simulink model "Standalone_SpeedControl"  (R2023b)
settings: Solver=FixedStepAuto  StartTime=0.0  StopTime=Inf  RelTol=1e-3  EnableMultiTasking=on
undefined symbols (not defined in the file): SensorCurrent_VoltAtZero, SensorCurrent_VoltPerAmp
libraries: mcbpositiondecoderlib x1
settings Model: DataDictionary=Data_GeneralDefinition.sldd  SimulationMode=external  ExtModeTrigDuration=20  Creator=rodri  LastModifiedBy=rodri
settings OptimizationCC: DefaultUnderspecifiedDataType=single  EnhancedBackFolding=on  PassReuseOutputArgsAs=Individual arguments  MaxStackSize=1024  OptimizeBlockOrder=speed  DifferentSizesBufferReuse=on  EfficientTunableParamExpr=on
settings DebuggingCC: ParameterTunabilityLossMsg=error
settings HardwareCC: ProdBitPerChar=16  ProdBitPerInt=16  ProdBitPerPointer=32  ProdBitPerSizeT=32  ProdBitPerPtrDiffT=32  ProdLargestAtomicInteger=Integer  ProdLargestAtomicFloat=None  ProdWordSize=16  ProdLongLongMode=on  ProdHWDeviceType=Texas Instruments->C2000  HardwareBoardFeatureSet=SoCBlockset
settings ModelReferenceCC: EnableParallelModelReferenceBuilds=on  ModelReferenceNumInstancesAllowed=Single
settings SFSimCC: MATLABDynamicMemAlloc=off
settings RTWCC: Description=Embedded Coder  SystemTargetFile=ert.tlc  HardwareBoard=TI Piccolo F28069M LaunchPad  TemplateMakefile=ert_default_tmf  Toolchain=Texas Instruments Code Composer Studio (C2000)  CodeProfilingSaveOptions=MetricsOnly
settings CodeAppCC: ForceParamTrailComments=on  IgnoreCustomStorageClasses=off  OperatorAnnotations=on  SimulinkDataObjDesc=on  SFDataObjDesc=on  InsertBlockDesc=on
settings ERTTargetCC: CodeReplacementLibrary=TI C28x  ExtMode=on  ExtModeTransport=4  ExtModeStaticAlloc=on  ExtModeAutomaticAllocSize=off  ExtModeStaticAllocSize=2000  ExtModeMexFile=ext_xcp  ExtModeMexArgs=1 4 115200  ExtModeIntrfLevel=Level2 - Open

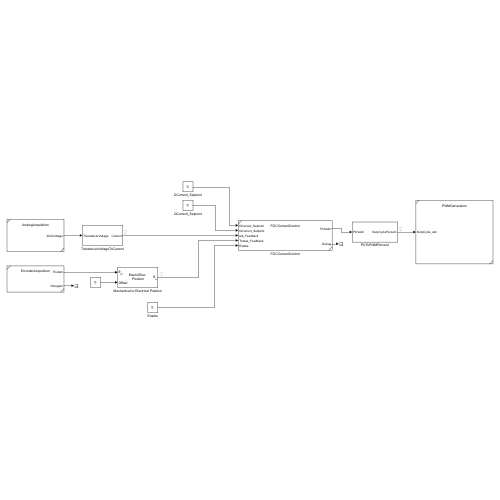
[thumbnail: Simulink's stored preview of the top-level diagram]
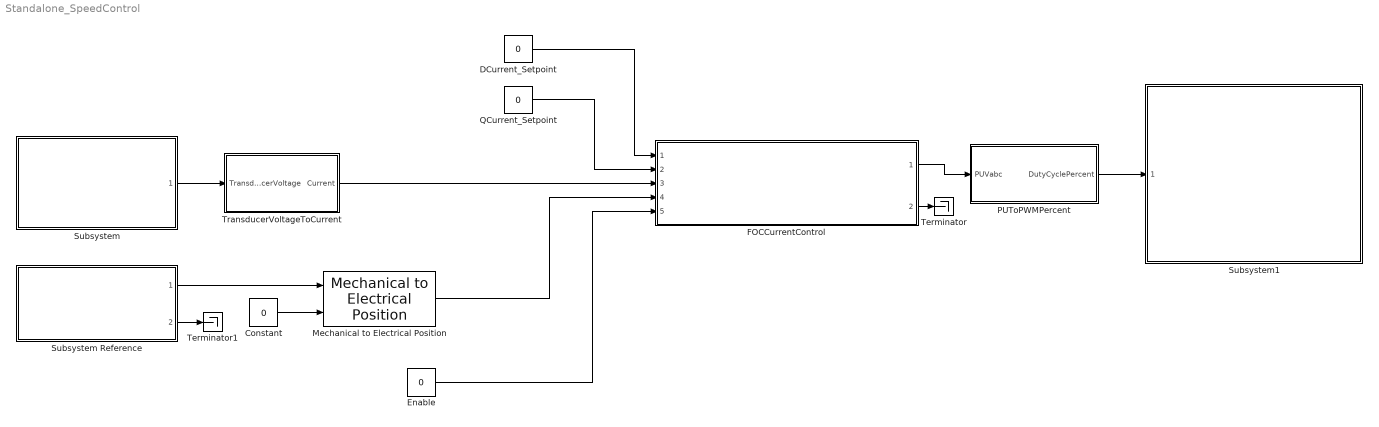
== system Standalone_SpeedControl ==
  Constant : Constant  Value=0
  DCurrent_Setpoint : Constant  Value=0  OutDataTypeStr=single
  Enable : Constant  Value=0
  FOCCurrentControl : Subsystem  ReferencedSubsystem=FOCCurrentControl
  Mechanical to Electrical Position : mcbpositiondecoderlib/Mechanical to Electrical Position  PolePairsInputType=Specify via dialog  NrPP=5  selectedRange=Radians  MechOfstInputType=Input port  mechOffsetIn=0  maxAngleIn=2*pi  InputDataType=single  VariantSelect=floating-point
      settings: LibrarySourceBlock=mcblib/Sensor Decoders/Mechanical to Electrical Position
  PUToPWMPercent : Subsystem
  QCurrent_Setpoint : Constant  Value=0  OutDataTypeStr=single
  Subsystem : Subsystem  ReferencedSubsystem=AnalogAcquisition
  Subsystem Reference : Subsystem  ReferencedSubsystem=EncoderAcquisition
  Subsystem1 : Subsystem  ReferencedSubsystem=PWMGeneration
  Terminator : Terminator
  Terminator1 : Terminator
  TransducerVoltageToCurrent : Subsystem
  wires:
  Subsystem/1 -> TransducerVoltageToCurrent/1(TransducerVoltage)
  PUToPWMPercent/1(DutyCyclePercent) -> Subsystem1/1
  TransducerVoltageToCurrent/1(Current) -> FOCCurrentControl/3
  DCurrent_Setpoint/1 -> FOCCurrentControl/1
  QCurrent_Setpoint/1 -> FOCCurrentControl/2
  Mechanical to Electrical Position/1 -> FOCCurrentControl/4
  FOCCurrentControl/1 -> PUToPWMPercent/1(PUVabc)
  Enable/1 -> FOCCurrentControl/5
  FOCCurrentControl/2 -> Terminator/1
  Subsystem Reference/1 -> Mechanical to Electrical Position/1
  Subsystem Reference/2 -> Terminator1/1
  Constant/1 -> Mechanical to Electrical Position/2

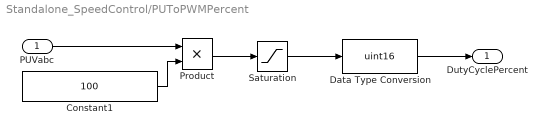
== system Standalone_SpeedControl/PUToPWMPercent ==
  PUVabc : Inport
  Constant1 : Constant  Value=100  OutDataTypeStr=Inherit: Inherit via back propagation  SampleTime=-1
  Data Type Conversion : DataTypeConversion  OutDataTypeStr=uint16  SaturateOnIntegerOverflow=off  RndMeth=Floor
  Product : Product  OutDataTypeStr=Inherit: Inherit via back propagation
  Saturation : Saturate  UpperLimit=100  LowerLimit=0
  DutyCyclePercent : Outport
  wires:
  Constant1/1 -> Product/2
  PUVabc/1 -> Product/1
  Saturation/1 -> Data Type Conversion/1
  Data Type Conversion/1 -> DutyCyclePercent/1
  Product/1 -> Saturation/1

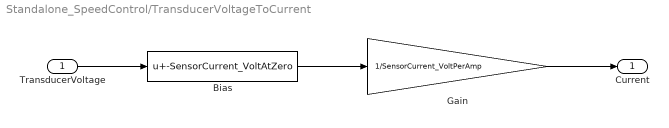
== system Standalone_SpeedControl/TransducerVoltageToCurrent ==
  TransducerVoltage : Inport
  Bias : Bias  Bias=-SensorCurrent_VoltAtZero  SaturateOnIntegerOverflow=off
  Gain : Gain  Gain=1/SensorCurrent_VoltPerAmp
  Current : Outport
  wires:
  Gain/1 -> Current/1
  TransducerVoltage/1 -> Bias/1
  Bias/1 -> Gain/1
